simulink model "IntelligentCruiseControl"  (R2022b)
settings: Solver=ode1  StartTime=0.0  StopTime=600  FixedStep=0.1  RelTol=1e-3  EnableMultiTasking=on
InitFcn:
  | IntelligentCruiseControlMenu
StopFcn:
  | IntelligentCruiseControlAutoGrading
values from neighbouring files (symbols this model uses):
  choice = menu('Types of Controllers',                  'Velocity Controller',              	'Headway Controller',                 'Intelligent Cruise Controller')    [IntelligentCruiseControlMenu.m]
libraries: simulink x2
settings Model: Creator=burl  LastModifiedBy=prajw
settings SolverCC: AlgebraicLoopSolver=TrustRegion
settings DataIOCC: LimitDataPoints=on  SaveFormat=Array  SignalLoggingSaveFormat=ModelDataLogs  ReturnWorkspaceOutputs=off
settings OptimizationCC: BlockReduction=off  OptimizeBlockIOStorage=off  BufferReuse=off  GlobalBufferReuse=off  ExpressionFolding=off  LocalBlockOutputs=off  LifeSpan=inf  OptimizeDataStoreBuffers=off  BusAssignmentInplaceUpdate=off
settings DebuggingCC: UnderspecifiedInitializationDetection=Classic  MergeDetectMultiDrivingBlocksExec=none  SolverPrmCheckMsg=warning  MultiTaskDSMMsg=warning  MultiTaskCondExecSysMsg=none  UnconnectedInputMsg=warning  UnconnectedOutputMsg=warning  UnconnectedLineMsg=warning  StateNameClashWarn=warning  PregeneratedLibrarySubsystemCodeDiagnostic=none  SFUnexpectedBacktrackingDiag=warning  SFNoUnconditionalDefaultTransitionDiag=warning  SFExecutionAtInitializationDiag=none  SFMachineParentedDataDiag=warning  ArithmeticOperatorsInVariantConditions=warning
settings HardwareCC: ProdBitPerPointer=32  ProdBitPerSizeT=32  ProdBitPerPtrDiffT=32  ProdLargestAtomicFloat=None  ProdWordSize=32  ProdHWDeviceType=Generic->Custom  TargetIntDivRoundTo=Zero  TargetEndianess=LittleEndian  TargetHWDeviceType=Generic->Custom
settings ModelReferenceCC: EnableRefExpFcnMdlSchedulingChecks=on  PropagateSignalLabelsOutOfModel=off
settings SFSimCC: SimUseLocalCustomCode=off  CustomCodeUndefinedFunction=UseInterfaceOnly
settings RTWCC: Description=dSPACE DS1006 Hardware Platform  SystemTargetFile=rti1006.tlc  MakeCommand=make_rti  TemplateMakefile=rti1006.tmf  RTWUseLocalCustomCode=off
settings CodeAppCC: StateflowObjectComments=on
settings STFCustomTargetCC: ParMdlRefBuildCompliant=on  MatFileLogging=on  CPPClassGenCompliant=on  GRTInterface=on  SystemTargetFile=rti1006.tlc
settings GRTTargetCC: TargetLangStandard=C89/C90 (ANSI)  CompOptLevelCompliant=off  ConcurrentExecutionCompliant=off  CombineOutputUpdateFcns=off  GRTInterface=on  UseToolchainInfoCompliant=off
settings ConfigComp: CovMetricSettings=dw  CovSaveCumulativeToWorkspaceVar=on  CovSaveSingleToWorkspaceVar=on  CovExternalEMLEnable=off

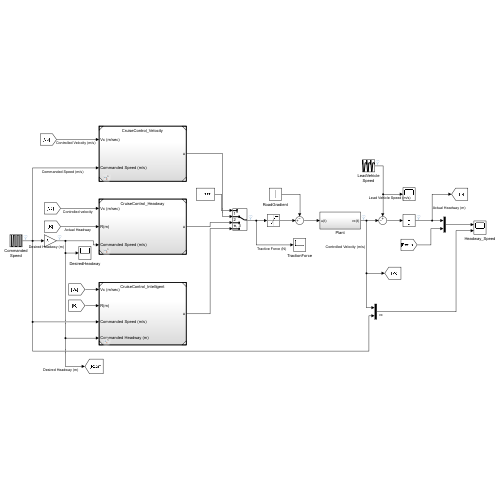
[thumbnail: Simulink's stored preview of the top-level diagram]
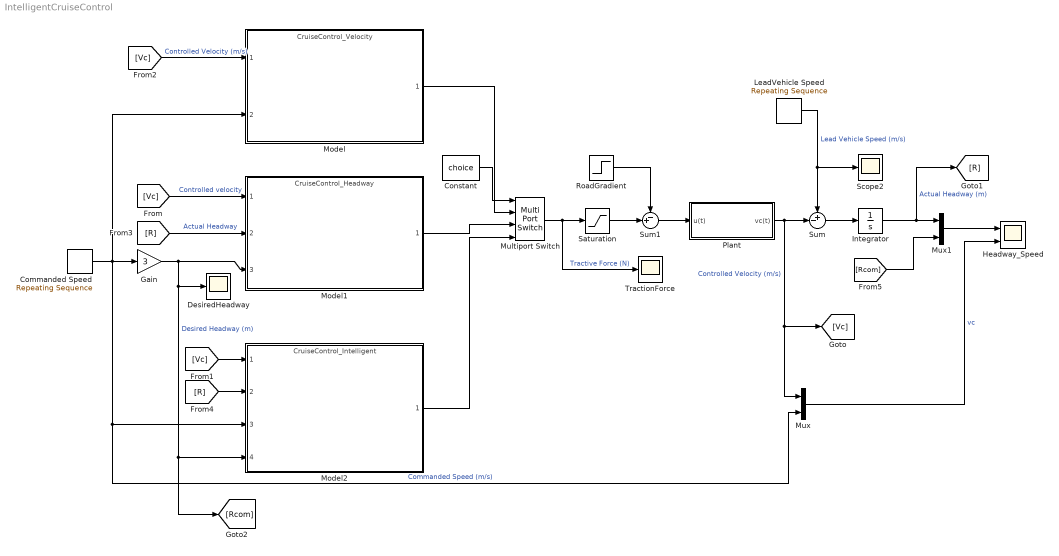
== system IntelligentCruiseControl ==
  Commanded Speed : simulink/Sources/Repeating Sequence  rep_seq_t=[0 100 110 400 410 600]  rep_seq_y=[27 27 25 25 27 27]
  Constant : Constant  Value=choice
  DesiredHeadway : Scope
  Gain : Gain  Gain=3
  Headway_Speed : Scope  NumInputPorts=2
  Integrator : Integrator  InitialCondition=81
  LeadVehicle Speed : simulink/Sources/Repeating Sequence  rep_seq_t=[0 30 150 250 350 600]  rep_seq_y=[27 30 22 22 28 28]
  Model : ModelReference  ModelNameDialog=CruiseControl_Velocity  SimulationMode=Normal  ModelReferenceVersion=9.13
  Model1 : ModelReference  ModelNameDialog=CruiseControl_Headway  SimulationMode=Normal  ModelReferenceVersion=9.2
  Model2 : ModelReference  ModelNameDialog=CruiseControl_Intelligent  SimulationMode=Normal  ModelReferenceVersion=10.0
  Multiport Switch : MultiPortSwitch  SaturateOnIntegerOverflow=off  InputSameDT=off
  Mux : Mux  Inputs=2
  Mux1 : Mux  Inputs=2
  Plant : Subsystem
  RoadGradient : Step  Time=500  After=500  SampleTime=0
  Saturation : Saturate  UpperLimit=1e7  LowerLimit=-1e7
  Scope2 : Scope
  Sum : Sum  Inputs=+-|
  Sum1 : Sum  Inputs=-+|
  TractionForce : Scope
  wires:
  Sum/1 -> Integrator/1
  Integrator/1 -> Mux1/1, [R]  "Actual Headway (m)"
  LeadVehicle Speed/1 -> Scope2/1, Sum/1  "Lead Vehicle Speed (m/s)"
  RoadGradient/1 -> Sum1/1
  Sum1/1 -> Plant/1(u(t))
  Plant/1(vc(t)) -> Mux/1, [Vc], Sum/2  "Controlled Velocity (m/s)"
  Model/1 -> Multiport Switch/2
  Commanded Speed/1 -> Model/2, Gain/1, Mux/2, Model2/3  "Commanded Speed (m/s)"
  [Vc] -> Model1/1  "Controlled velocity"
  [Vc] -> Model2/1
  [Vc] -> Model/1  "Controlled Velocity (m/s)"
  [R] -> Model1/2  "Actual Headway"
  [R] -> Model2/2
  Mux/1 -> Headway_Speed/2  "vc"
  Model1/1 -> Multiport Switch/3
  Model2/1 -> Multiport Switch/4
  Multiport Switch/1 -> TractionForce/1, Saturation/1  "Tractive Force (N)"
  Constant/1 -> Multiport Switch/1
  Saturation/1 -> Sum1/2
  Gain/1 -> Model1/3, [Rcom], Model2/4, DesiredHeadway/1  "Desired Headway (m)"
  [Rcom] -> Mux1/2
  Mux1/1 -> Headway_Speed/1

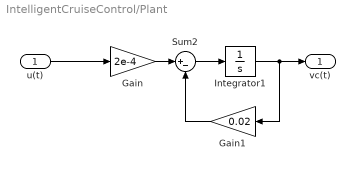
== system IntelligentCruiseControl/Plant ==
  u(t) : Inport
  Gain : Gain  Gain=2e-4
  Gain1 : Gain  Gain=0.02
  Integrator1 : Integrator  InitialCondition=27
  Sum2 : Sum  Inputs=|+-
  vc(t) : Outport  VectorParamsAs1DForOutWhenUnconnected=off
  wires:
  Gain/1 -> Sum2/1
  Sum2/1 -> Integrator1/1
  Gain1/1 -> Sum2/2
  Integrator1/1 -> Gain1/1, vc(t)/1
  u(t)/1 -> Gain/1
